simulink model "monteCarloPMSMsim"  (R2022b)
settings: Solver=VariableStepAuto  StartTime=0.0  StopTime=simParam.stopTime  FixedStep=simParam.maxStep  MaxStep=simParam.maxStep  RelTol=1e-3
values from neighbouring files (symbols this model uses):
  aug =     [controllerGains.mat]
  B = noise.param.B(i)    [monteCarloPMSM.m]
  J = noise.param.J(i)    [monteCarloPMSM.m]
  lambdaM = noise.param.lambdaM(i)    [monteCarloPMSM.m]
  Ld = noise.param.Ld(i)    [monteCarloPMSM.m]
  Lq = noise.param.Lq(i)    [monteCarloPMSM.m]
  N = 18    [monteCarloPMSM.m]
  opPoint =     [controllerGains.mat]
  Rs = noise.param.Rs(i)    [monteCarloPMSM.m]
  var_disturbance = [48 48]*10e-9    [monteCarloPMSM.m]
  var_noise = [10 10 100]*10e-11    [monteCarloPMSM.m]
undefined symbols (not defined in the file or in its folder): simParam, X_i
settings Model: Creator=kaike  LastModifiedBy=kaike

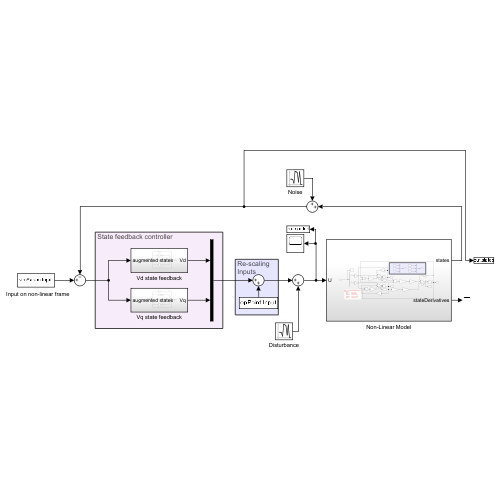
[thumbnail: Simulink's stored preview of the top-level diagram]
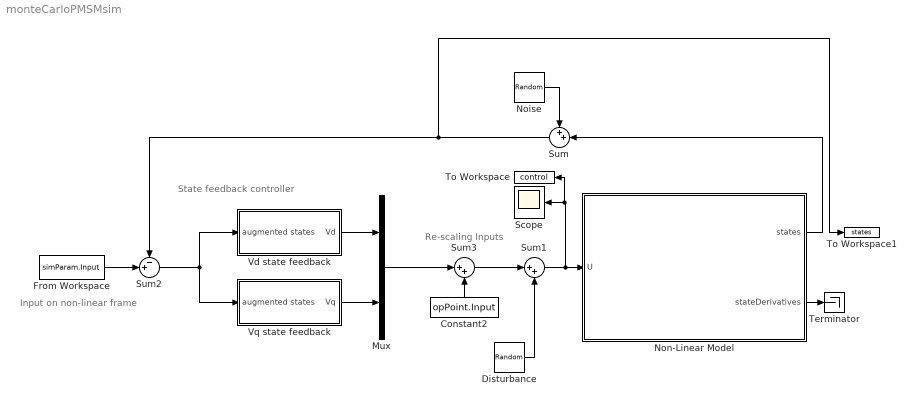
== system monteCarloPMSMsim ==
  note: Re-scaling
      | Inputs
  note: Input on non-linear frame
  note: State feedback controller
  Constant2 : Constant  Value=opPoint.Input
  Disturbance : RandomNumber  Variance=var_disturbance  Seed=simParam.seed(2)
  From Workspace : FromWorkspace  VariableName=simParam.Input  OutputAfterFinalValue=Holding final value
  Mux : Mux  Inputs=2
  Noise : RandomNumber  Variance=var_noise  Seed=simParam.seed(1)
  "Non-Linear Model " : Subsystem
  Scope : Scope
  Sum : Sum  Inputs=++|
  Sum1 : Sum  Inputs=|++
  Sum2 : Sum  Inputs=-+|
  Sum3 : Sum  Inputs=|++
  Terminator : Terminator
  To Workspace : ToWorkspace  VariableName=control  SampleTime=-1
  To Workspace1 : ToWorkspace  VariableName=states  SampleTime=-1
  Vd state feedback : Subsystem
  Vq state feedback : Subsystem
  wires:
  Mux/1 -> Sum3/1
  Constant2/1 -> Sum3/2
  Sum2/1 -> Vq state feedback/1(augmented states), Vd state feedback/1(augmented states)
  Vq state feedback/1(Vq) -> Mux/2
  Vd state feedback/1(Vd) -> Mux/1
  "Non-Linear Model "/1(states) -> Sum/2
  From Workspace/1 -> Sum2/2
  Sum/1 -> To Workspace1/1, Sum2/1
  Noise/1 -> Sum/1
  Sum1/1 -> Scope/1, To Workspace/1, "Non-Linear Model "/1(U)
  Sum3/1 -> Sum1/1
  Disturbance/1 -> Sum1/2
  "Non-Linear Model "/2(stateDerivatives) -> Terminator/1

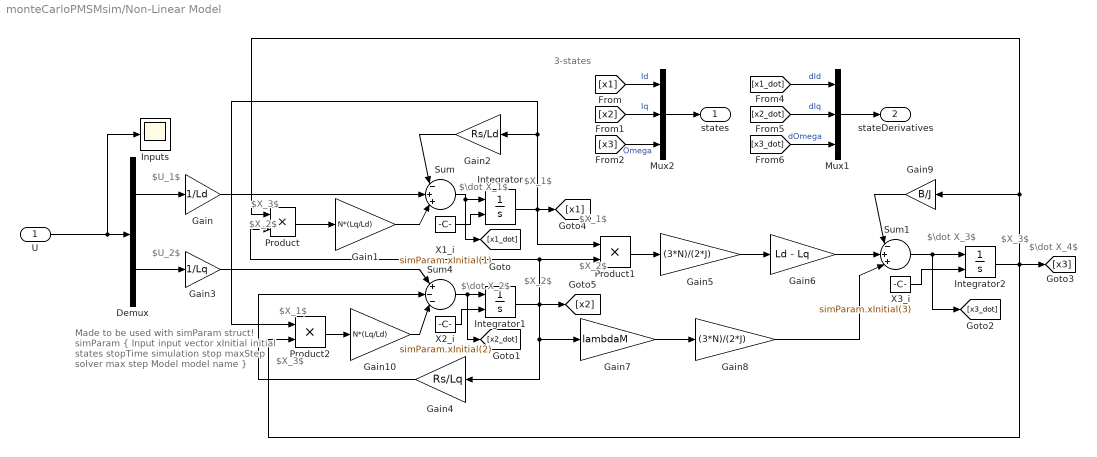
== system monteCarloPMSMsim/Non-Linear Model  ==
  note: $U_2$
  note: 3-states
  note: $X_2$
  note: $X_2$
  note: $X_3$
  note: $X_1$
  note: $X_1$
  note: $X_3$
  note: Made to be used with simParam struct!
      | simParam {
      | Input input vector
      | xInitial initial states
      | stopTime simulation stop
      | maxStep solver max step
      | Model model name
      | }
  note: $\dot X_3$
  note: $X_2$
  note: $X_1$
  note: $\dot X_2$
  note: $\dot X_4$
  note: $\dot X_1$
  note: $X_3$
  note: $U_1$
  U : Inport
  Demux : Demux  Outputs=2
  Gain : Gain  Gain=1/Ld
  Gain1 : Gain  Gain=N*(Lq/Ld)
  Gain10 : Gain  Gain=N*(Lq/Ld)
  Gain2 : Gain  Gain=Rs/Ld
  Gain3 : Gain  Gain=1/Lq
  Gain4 : Gain  Gain=Rs/Lq
  Gain5 : Gain  Gain=(3*N)/(2*J)
  Gain6 : Gain  Gain=Ld - Lq
  Gain7 : Gain  Gain=lambdaM
  Gain8 : Gain  Gain=(3*N)/(2*J)
  Gain9 : Gain  Gain=B/J
  Inputs : Scope
  Integrator : Integrator  InitialConditionSource=external  InitialCondition=simParam.X_initial(3)  ContinuousStateAttributes='Id'
  Integrator1 : Integrator  InitialConditionSource=external  InitialCondition=X_i(2)  ContinuousStateAttributes='Iq'
  Integrator2 : Integrator  InitialConditionSource=external  InitialCondition=10  ContinuousStateAttributes='omega'
  Mux1 : Mux  Inputs=3
  Mux2 : Mux  Inputs=3
  Product : Product
  Product1 : Product
  Product2 : Product
  Sum : Sum  Inputs=|-++|
  Sum1 : Sum  Inputs=|-++|
  Sum4 : Sum  Inputs=|+--|
  X1_i : Constant  Value=simParam.xInitial(1)  VectorParams1D=off
  X2_i : Constant  Value=simParam.xInitial(2)
  X3_i : Constant  Value=simParam.xInitial(3)
  states : Outport
  stateDerivatives : Outport  Port=2
  wires:
  Integrator/1 -> [x1], Product2/1, Gain2/1, Product1/1
  Sum4/1 -> [x2_dot], Integrator1/1
  [x1] -> Mux2/1  "Id"
  Integrator1/1 -> [x2], Product/2, Product1/2, Gain4/1, Gain7/1
  Gain/1 -> Sum/2
  Gain4/1 -> Sum4/2
  U/1 -> Inputs/1, Demux/1
  Demux/1 -> Gain/1
  Sum1/1 -> [x3_dot], Integrator2/1
  Integrator2/1 -> [x3], Product2/2, Gain9/1, Product/1
  Sum/1 -> [x1_dot], Integrator/1
  [x2_dot] -> Mux1/2  "dIq"
  Gain2/1 -> Sum/1
  Gain1/1 -> Sum/3
  Product1/1 -> Gain5/1
  X1_i/1 -> Integrator/2
  Gain3/1 -> Sum4/1
  Product/1 -> Gain1/1
  Gain7/1 -> Gain8/1
  Gain5/1 -> Gain6/1
  [x1_dot] -> Mux1/1  "dId"
  [x2] -> Mux2/2  "Iq"
  [x3] -> Mux2/3  "Omega"
  [x3_dot] -> Mux1/3  "dOmega"
  Gain9/1 -> Sum1/1
  Product2/1 -> Gain10/1
  X3_i/1 -> Integrator2/2
  Gain6/1 -> Sum1/2
  Demux/2 -> Gain3/1
  X2_i/1 -> Integrator1/2
  Mux2/1 -> states/1
  Gain8/1 -> Sum1/3
  Gain10/1 -> Sum4/3
  Mux1/1 -> stateDerivatives/1

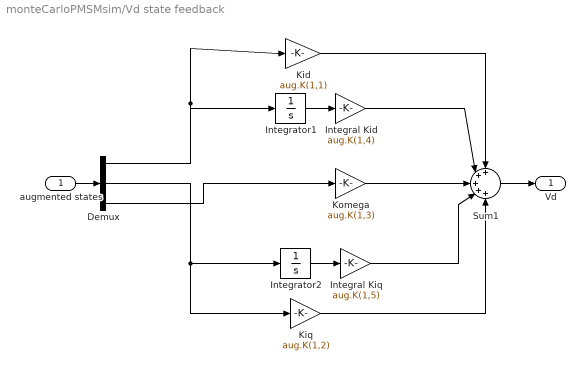
== system monteCarloPMSMsim/Vd state feedback ==
  augmented states : Inport
  Demux : Demux  Outputs=3
  Integral Kid : Gain  Gain=aug.K(1,4)
  Integral Kiq : Gain  Gain=aug.K(1,5)
  Integrator1 : Integrator
  Integrator2 : Integrator
  Kid : Gain  Gain=aug.K(1,1)
  Kiq : Gain  Gain=aug.K(1,2)
  Komega : Gain  Gain=aug.K(1,3)
  Sum1 : Sum  Inputs=+++++
  Vd : Outport
  wires:
  augmented states/1 -> Demux/1
  Integrator1/1 -> Integral Kid/1
  Sum1/1 -> Vd/1
  Integrator2/1 -> Integral Kiq/1
  Demux/1 -> Kid/1, Integrator1/1
  Integral Kid/1 -> Sum1/2
  Kid/1 -> Sum1/1
  Demux/3 -> Komega/1
  Komega/1 -> Sum1/3
  Demux/2 -> Kiq/1, Integrator2/1
  Integral Kiq/1 -> Sum1/4
  Kiq/1 -> Sum1/5

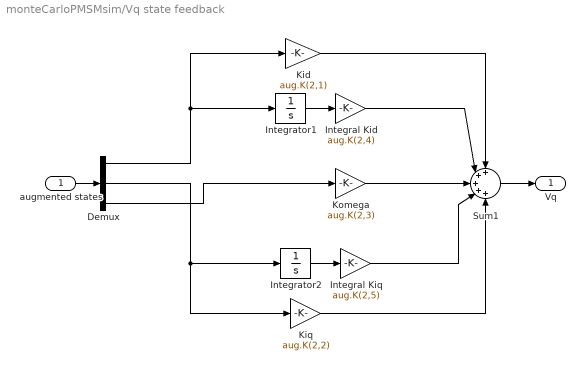
== system monteCarloPMSMsim/Vq state feedback ==
  augmented states : Inport
  Demux : Demux  Outputs=3
  Integral Kid : Gain  Gain=aug.K(2,4)
  Integral Kiq : Gain  Gain=aug.K(2,5)
  Integrator1 : Integrator
  Integrator2 : Integrator
  Kid : Gain  Gain=aug.K(2,1)
  Kiq : Gain  Gain=aug.K(2,2)
  Komega : Gain  Gain=aug.K(2,3)
  Sum1 : Sum  Inputs=+++++
  Vq : Outport
  wires:
  augmented states/1 -> Demux/1
  Integrator1/1 -> Integral Kid/1
  Sum1/1 -> Vq/1
  Integrator2/1 -> Integral Kiq/1
  Demux/1 -> Kid/1, Integrator1/1
  Integral Kid/1 -> Sum1/2
  Kid/1 -> Sum1/1
  Demux/3 -> Komega/1
  Komega/1 -> Sum1/3
  Demux/2 -> Kiq/1, Integrator2/1
  Integral Kiq/1 -> Sum1/4
  Kiq/1 -> Sum1/5
